simulink model "sim_test_model"  (R2019b)
settings: Solver=VariableStepAuto  StartTime=0.0  StopTime=10.0  RelTol=1e-3
values from neighbouring files (symbols this model uses):
  Ts = 0.2    [test_run_simulation.m]
libraries: simulink x1
settings Model: Creator=billtubbs  LastModifiedBy=billtubbs

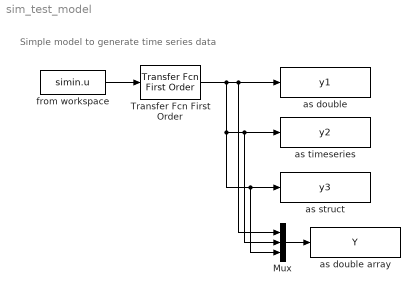
== system sim_test_model ==
  note: Simple model to generate time series data
  Mux : Mux  Inputs=3
  Transfer Fcn First Order : simulink/Discrete/Transfer Fcn First Order  PoleZ=0.9  ICPrevOutput=0.0  DoSatur=off
      settings: SourceProductName=Simulink
  as double : ToWorkspace  VariableName=y1  SampleTime=Ts
  as double array : ToWorkspace  VariableName=Y  SampleTime=Ts
      settings: Save2DSignal=2-D array (concatenate along first dimension)
  as struct : ToWorkspace  VariableName=y3  SaveFormat=Structure With Time  SampleTime=Ts
  as timeseries : ToWorkspace  VariableName=y2  SaveFormat=Timeseries  SampleTime=Ts
  from workspace : FromWorkspace  VariableName=simin.u  SampleTime=0
  wires:
  from workspace/1 -> Transfer Fcn First Order/1
  Transfer Fcn First Order/1 -> Mux/1, as double/1, Mux/2, as timeseries/1, Mux/3, as struct/1
  Mux/1 -> as double array/1
